simulink model "Investigation_ASM"  (R2020a)
settings: Solver=ode5  StartTime=0.0  StopTime=t_end  FixedStep=dt  RelTol=1e-3
values from neighbouring files (symbols this model uses):
  dt = 1e-5    (= 1e-05)    [Experiment_3_ASM_Parameter.m]    (also in Experiment_3_PMSM_Parameter.m = 5e-06)
libraries: simulink x1
settings Model: Creator=julien  LastModifiedBy=ge29wel
settings DataIOCC: LimitDataPoints=on  SaveFormat=Array  ReturnWorkspaceOutputs=off
settings OptimizationCC: BlockReduction=off  BooleanDataType=off  LifeSpan=inf
settings DebuggingCC: SaveWithParameterizedLinksMsg=none  UnderspecifiedInitializationDetection=Classic  MergeDetectMultiDrivingBlocksExec=none  SignalResolutionControl=TryResolveAllWithWarning  SFUnexpectedBacktrackingDiag=warning  SFNoUnconditionalDefaultTransitionDiag=warning  SFExecutionAtInitializationDiag=none  ArithmeticOperatorsInVariantConditions=warning
settings HardwareCC: ProdBitPerPointer=32  ProdBitPerSizeT=32  ProdBitPerPtrDiffT=32  ProdLargestAtomicFloat=None  ProdIntDivRoundTo=Undefined  ProdEndianess=Unspecified  ProdWordSize=32  ProdHWDeviceType=32-bit Generic  TargetUnknown=on
settings ModelReferenceCC: PropagateSignalLabelsOutOfModel=off
settings SFSimCC: SimUseLocalCustomCode=off  CustomCodeUndefinedFunction=UseInterfaceOnly
settings RTWCC: RTWUseLocalCustomCode=off
settings CodeAppCC: StateflowObjectComments=on
settings GRTTargetCC: TargetLangStandard=C89/C90 (ANSI)
settings ConfigComp: CovMetricSettings=dw  CovHtmlReporting=on  CovSaveCumulativeToWorkspaceVar=on  CovSaveSingleToWorkspaceVar=on  CovExternalEMLEnable=off  CovSFcnEnable=off

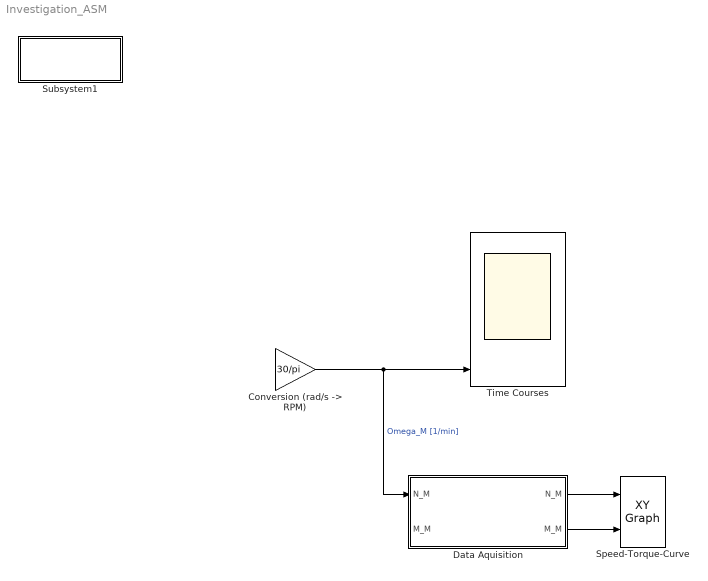
== system Investigation_ASM ==
  "Conversion (rad/s -> RPM)" : Gain  Gain=30/pi
  Data Aquisition : Subsystem  mask{downsampling=100}
  Speed-Torque-Curve : simulink/Sinks/XY Graph  xmin=-1  xmax=3500  ymin=-10  ymax=35  st=-1
  Subsystem1 : Subsystem
      settings: OpenFcn=Experiment_3_ASM_Parameter
      mask Display: disp('Initialize\n (doppelklicken)')
  Time Courses : Scope  NumInputPorts=4
  wires:
  "Conversion (rad/s -> RPM)"/1 -> Data Aquisition/1(N_M), Time Courses/4  "Omega_M [1/min]"
  ? -> Data Aquisition/2(M_M), Time Courses/3  "M_M [Nm]"
  ? -> Time Courses/2  "i_r^r [A]"
  ? -> Time Courses/1  "i_s^s [A]"
  ? -> "Conversion (rad/s -> RPM)"/1
  Data Aquisition/2("M_M ") -> Speed-Torque-Curve/2
  Data Aquisition/1("N_M ") -> Speed-Torque-Curve/1

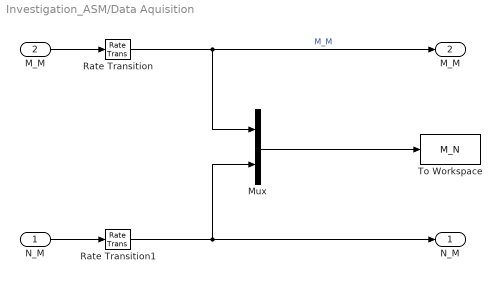
== system Investigation_ASM/Data Aquisition ==
  N_M : Inport
  M_M : Inport  Port=2
  Mux : Mux  Inputs=2
  Rate Transition : RateTransition  OutPortSampleTime=downsampling*dt
  Rate Transition1 : RateTransition  OutPortSampleTime=downsampling*dt
  To Workspace : ToWorkspace  VariableName=M_N  SaveFormat=Structure  SampleTime=-1
  "N_M " : Outport
  "M_M " : Outport  Port=2
  wires:
  Mux/1 -> To Workspace/1
  Rate Transition/1 -> Mux/1, "M_M "/1  "M_M"
  Rate Transition1/1 -> Mux/2, "N_M "/1
  N_M/1 -> Rate Transition1/1
  M_M/1 -> Rate Transition/1

== system Investigation_ASM/Subsystem1 ==
